simulink model "withDOB"  (R2017a)
settings: Solver=VariableStepAuto  StartTime=0.0  StopTime=10.0  RelTol=1e-3
values from neighbouring files (symbols this model uses):
  Gd1 = c2d(sysu2y,0.01)    [HW03.m]
undefined symbols (not defined in the file or in its folder): Z
libraries: cstblocks x3
settings Model: Creator=15062  LastModifiedBy=15062

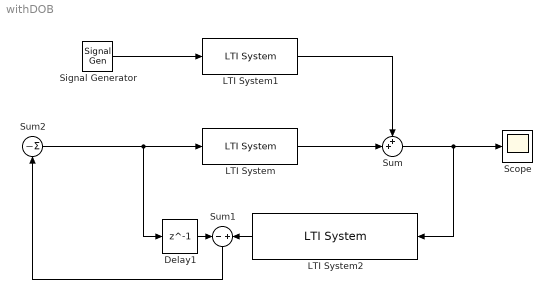
== system withDOB ==
  Delay1 : Delay  DelayLength=1  SampleTime=0.01
  LTI System : cstblocks/LTI System  sys=Gd1  IC=[]
  LTI System1 : cstblocks/LTI System  sys=Gd2  IC=[]
  LTI System2 : cstblocks/LTI System  sys=Gd1^(-1)*Z^(-1)  IC=[]
  Scope : Scope
  Signal Generator : SignalGenerator  Units=rad/sec
  Sum : Sum  Inputs=++|
  Sum1 : Sum  Inputs=-|+
  Sum2 : Sum  Inputs=|-
  wires:
  LTI System1/1 -> Sum/1
  Sum2/1 -> Delay1/1, LTI System/1
  Signal Generator/1 -> LTI System1/1
  LTI System/1 -> Sum/2
  Sum/1 -> LTI System2/1, Scope/1
  Delay1/1 -> Sum1/1
  LTI System2/1 -> Sum1/2
  Sum1/1 -> Sum2/1
